simulink model "gm_Controller"  (R2016b)
settings: Solver=FixedStepAuto  StartTime=0.0  StopTime=256  FixedStep=1  RelTol=1e-3
settings Model: Creator=Arthur  LastModifiedBy=Arthur
settings DataIOCC: SaveOutput=off  SaveTime=off
settings OptimizationCC: BlockReduction=off  ConditionallyExecuteInputs=off  DefaultParameterBehavior=Inlined
settings DebuggingCC: InheritedTsInSrcMsg=none  StrictBusMsg=ErrorOnBusTreatedAsVector

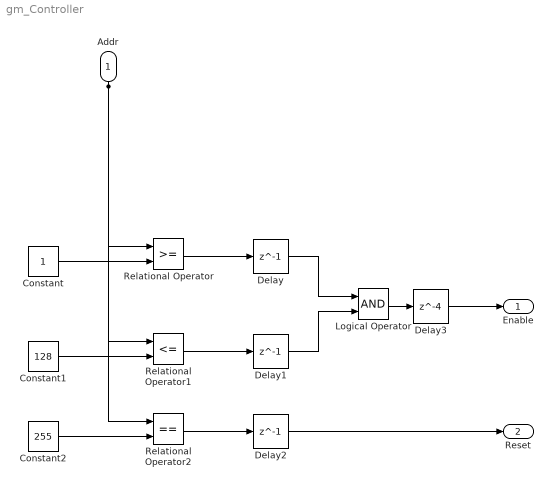
== system gm_Controller ==
  Addr : Inport  OutDataTypeStr=fixdt(1,17,0)  PortDimensions=1  SampleTime=1
  Constant : Constant  OutDataTypeStr=fixdt(0,10,0)
  Constant1 : Constant  Value=128  OutDataTypeStr=fixdt(0,10,0)
  Constant2 : Constant  Value=255  OutDataTypeStr=fixdt(0,10,0)
  Delay : Delay  DelayLength=1
  Delay1 : Delay  DelayLength=1
  Delay2 : Delay  DelayLength=1
  Delay3 : Delay  DelayLength=4
  Logical Operator : Logic  AllPortsSameDT=off  OutDataTypeStr=boolean
  Relational Operator : RelationalOperator  OutDataTypeStr=boolean  RndMeth=Simplest
  Relational Operator1 : RelationalOperator  Operator=<=  OutDataTypeStr=boolean  RndMeth=Nearest
  Relational Operator2 : RelationalOperator  Operator===  OutDataTypeStr=boolean  RndMeth=Simplest
  Enable : Outport  OutDataTypeStr=boolean  PortDimensions=1  SampleTime=[1,0]
  Reset : Outport  Port=2  OutDataTypeStr=boolean  PortDimensions=1  SampleTime=[1,0]
  wires:
  Addr/1 -> Relational Operator2/1, Relational Operator1/1, Relational Operator/1
  Constant/1 -> Relational Operator/2
  Constant1/1 -> Relational Operator1/2
  Constant2/1 -> Relational Operator2/2
  Delay/1 -> Logical Operator/1
  Delay1/1 -> Logical Operator/2
  Delay2/1 -> Reset/1
  Delay3/1 -> Enable/1
  Logical Operator/1 -> Delay3/1
  Relational Operator/1 -> Delay/1
  Relational Operator1/1 -> Delay1/1
  Relational Operator2/1 -> Delay2/1
